simulink model "Demo3_model3"  (R2025b)
settings: Solver=VariableStepAuto  StartTime=0.0  StopTime=10.0  RelTol=1e-3
settings Model: Creator=FilipBabiec  LastModifiedBy=FilipBabiec

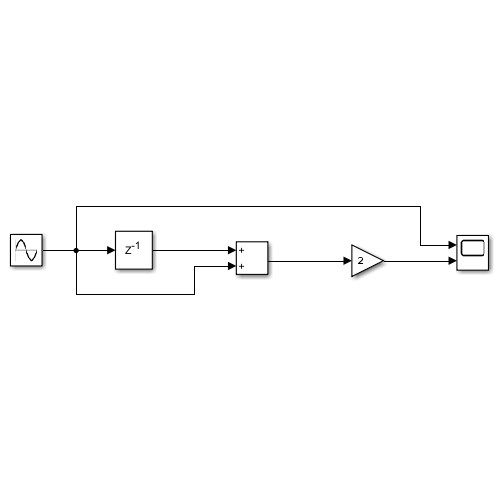
[thumbnail: Simulink's stored preview of the top-level diagram]
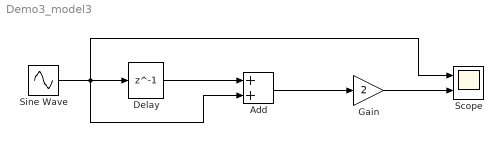
== system Demo3_model3 ==
  Add : Sum
  Delay : Delay  DelayLength=1  InputProcessing=Columns as channels (frame based)
  Gain : Gain  Gain=2
  Scope : Scope  NumInputPorts=2
      settings: ActiveDisplayYMinimum=-4.9741505260554328  ActiveDisplayYMaximum=4.9702424851127969
  Sine Wave : Sin  SampleTime=0
  wires:
  Sine Wave/1 -> Scope/1, Add/2, Delay/1
  Delay/1 -> Add/1
  Add/1 -> Gain/1
  Gain/1 -> Scope/2
